simulink model "dynamic_controller_system"  (R2014b)
settings: Solver=ode3  StartTime=0.0  StopTime=tfinal  FixedStep=Tsample  RelTol=2e-3
libraries: Controllers x5, simulink x4, DiffSteer_model x2
settings Model: Creator=Felipe  LastModifiedBy=Martins
settings DataIOCC: MaxDataPoints=10000
settings DebuggingCC: UnderspecifiedInitializationDetection=Classic  MergeDetectMultiDrivingBlocksExec=none  SolverPrmCheckMsg=none  StateNameClashWarn=warning

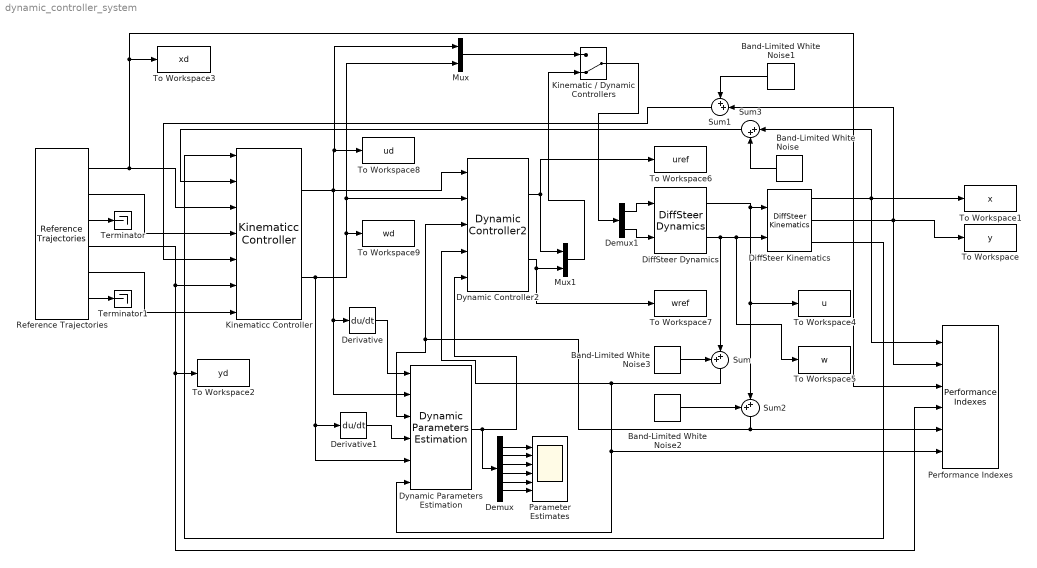
== system dynamic_controller_system ==
  Band-Limited White Noise : simulink/Sources/Band-Limited White Noise  Cov=[0.00001]  Ts=0.1  seed=[23341]
  Band-Limited White Noise1 : simulink/Sources/Band-Limited White Noise  Cov=[0.00001]  Ts=0.1  seed=[20001]
  Band-Limited White Noise2 : simulink/Sources/Band-Limited White Noise  Cov=[0.00002]  Ts=0.1  seed=[11141]
  Band-Limited White Noise3 : simulink/Sources/Band-Limited White Noise  Cov=[0.00002]  Ts=0.1  seed=[01234]
  Demux : Demux  Outputs=6
  Demux1 : Demux  Outputs=2
  Derivative : Derivative
  Derivative1 : Derivative
  DiffSteer Dynamics : DiffSteer_model/DiffSteer Dynamics  umax=0.75  wmax=1.745  dumax=0.3  dwmax=1.745  param=[0.2604 0.2509 -0.000499 0.9965 0.00263 1.0768]
  DiffSteer Kinematics : DiffSteer_model/DiffSteer Kinematics  x0=[0.2, 0, 0]  a=0.2  umax=0.75  wmax=1.745  dumax=0.3  dwmax=1.745
  Dynamic Parameters Estimation : Controllers/Dynamic Parameters Estimation  ku=4  kw=4  lu=1  lw=1  inicia_adapt=inicia_adapt  theta=[0.2604 0.2509 -0.000499 0.9965 0.00263 1.0768]/1.5  gamma=[1.7 1.1 0.5 0.3 0.01 0.5]  sig_mod=[0.0005 0.001 0.001 0.00006 0.001 0.001]
  Dynamic Controller2 : Controllers/Dynamic  Controller2  ku=4  kw=4  lu=1  lw=1
  Kinematic / Dynamic Controllers : ManualSwitch  CurrentSetting=0
  Kinematicc Controller : Controllers/Kinematicc Controller  kx=0.1  ky=0.1  lx=0.1  ly=0.1  a=0.2
  Mux : Mux  Inputs=2
  Mux1 : Mux  Inputs=2
  Parameter Estimates : Scope  NumInputPorts=6
      settings: TimeRange=250  YMin=0~0~-1~0~-0.5~0  YMax=10~15~0~6~1~10
  Performance Indexes : Controllers/Performance  Indexes
  Reference Trajectories : Controllers/Reference Trajectories  trajectory_type=2  wf=0.25  raio_ref_1=1  delta_raio=-0.1  t_delta_raio=60  xd=[1, -2]
  Sum : Sum  Inputs=++|
  Sum1 : Sum  Inputs=++|
  Sum2 : Sum  Inputs=++|
  Sum3 : Sum  Inputs=|++
  Terminator : Terminator
  Terminator1 : Terminator
  To Workspace : ToWorkspace  VariableName=y  SampleTime=-1
  To Workspace1 : ToWorkspace  VariableName=x  SampleTime=-1
  To Workspace2 : ToWorkspace  VariableName=yd  SampleTime=-1
  To Workspace3 : ToWorkspace  VariableName=xd  SampleTime=-1
  To Workspace4 : ToWorkspace  VariableName=u  SampleTime=-1
  To Workspace5 : ToWorkspace  VariableName=w  SampleTime=-1
  To Workspace6 : ToWorkspace  VariableName=uref  SampleTime=-1
  To Workspace7 : ToWorkspace  VariableName=wref  SampleTime=-1
  To Workspace8 : ToWorkspace  VariableName=ud  SampleTime=-1
  To Workspace9 : ToWorkspace  VariableName=wd  SampleTime=-1
  wires:
  Reference Trajectories/1 -> Performance Indexes/3, To Workspace3/1, Kinematicc Controller/3
  Reference Trajectories/2 -> Kinematicc Controller/4
  Reference Trajectories/4 -> Performance Indexes/4, To Workspace2/1, Kinematicc Controller/6
  Reference Trajectories/5 -> Kinematicc Controller/7
  DiffSteer Kinematics/1 -> Sum3/1, To Workspace1/1, Performance Indexes/1
  DiffSteer Kinematics/2 -> Sum1/2, To Workspace/1, Performance Indexes/2
  DiffSteer Kinematics/3 -> Kinematicc Controller/1
  Dynamic Parameters Estimation/1 -> Demux/1, Dynamic Controller2/5
  Kinematicc Controller/1 -> Dynamic Controller2/1, Mux/1, To Workspace8/1, Derivative/1, Dynamic Parameters Estimation/2
  Derivative/1 -> Dynamic Parameters Estimation/1
  Derivative1/1 -> Dynamic Parameters Estimation/4
  Reference Trajectories/3 -> Terminator/1
  Reference Trajectories/6 -> Terminator1/1
  DiffSteer Dynamics/2 -> Sum/2, To Workspace5/1, DiffSteer Kinematics/2
  Band-Limited White Noise3/1 -> Sum/1
  Sum/1 -> Dynamic Controller2/4, Performance Indexes/6, Dynamic Parameters Estimation/6
  DiffSteer Dynamics/1 -> To Workspace4/1, Sum2/2, DiffSteer Kinematics/1
  Band-Limited White Noise2/1 -> Sum2/1
  Sum2/1 -> Performance Indexes/5, Dynamic Controller2/3, Dynamic Parameters Estimation/3
  Band-Limited White Noise1/1 -> Sum1/1
  Band-Limited White Noise/1 -> Sum3/2
  Sum3/1 -> Kinematicc Controller/2
  Sum1/1 -> Kinematicc Controller/5
  Demux/6 -> Parameter Estimates/6
  Demux/5 -> Parameter Estimates/5
  Demux/4 -> Parameter Estimates/4
  Demux/3 -> Parameter Estimates/3
  Demux/2 -> Parameter Estimates/2
  Demux/1 -> Parameter Estimates/1
  Kinematicc Controller/2 -> Derivative1/1, Dynamic Parameters Estimation/5, Mux/2, Dynamic Controller2/2, To Workspace9/1
  Dynamic Controller2/1 -> Mux1/1, To Workspace6/1
  Dynamic Controller2/2 -> Mux1/2, To Workspace7/1
  Mux/1 -> Kinematic / Dynamic Controllers/1
  Kinematic / Dynamic Controllers/1 -> Demux1/1
  Demux1/2 -> DiffSteer Dynamics/2
  Demux1/1 -> DiffSteer Dynamics/1
  Mux1/1 -> Kinematic / Dynamic Controllers/2
